simulink model "gmStateSpaceHDL_buck_convert_test1_V2"  (R2025a)
settings: Solver=FixedStepDiscrete  StartTime=0.0  StopTime=0.005  FixedStep=1/40e6  RelTol=1e-3  AbsTol=1e-3
InitFcn:
  | load('C:\Users\bensa\Desktop\PI3_FPGA_BuckConverter\sschdl\buck_convert_test1\stateSpaceParameters.mat');
values from neighbouring files (symbols this model uses):
  stateSpaceParameters_1 =     [stateSpaceParameters.mat]
libraries: hdlsllib x4, hdlssclib x4, simulink x1
CloseFcn:
  | clear stateSpaceParameters_1
settings Model: Creator=bensa  LastModifiedBy=bensa
settings SolverCC: AutoScaleAbsTol=off  AlgebraicLoopSolver=TrustRegion  MaxZcPerStep=1.0
settings OptimizationCC: BlockReduction=off  ConditionallyExecuteInputs=off  DefaultParameterBehavior=Inlined
settings DebuggingCC: AlgebraicLoopMsg=error  SingleTaskRateTransMsg=error  UnconnectedInputMsg=warning  UnconnectedOutputMsg=warning  UnconnectedLineMsg=warning  SymbolicDimsDataTypeCodeGenerationDiagnostic=none
settings HardwareCC: ProdBitPerPointer=32.0  ProdBitPerSizeT=32.0  ProdBitPerPtrDiffT=32.0  ProdLargestAtomicFloat=None  ProdIntDivRoundTo=Undefined  ProdEndianess=Unspecified  ProdWordSize=32.0  ProdHWDeviceType=ASIC/FPGA->ASIC/FPGA  TargetBitPerPointer=64.0  TargetBitPerSizeT=64.0  TargetBitPerPtrDiffT=64.0  TargetLongLongMode=on  TargetIntDivRoundTo=Zero  TargetEndianess=LittleEndian  TargetWordSize=64.0  TargetHWDeviceType=Custom Processor->MATLAB Host Computer  ProdEqTarget=off
settings ModelReferenceCC: EnableRefExpFcnMdlSchedulingChecks=on
settings SFSimCC: CustomCodeUndefinedFunction=UseInterfaceOnly
settings RTWCC: GPUComputeCapability=3.5  DLArmComputeVersion=19.05
settings SimscapeCC: SimscapeLogType=all  SimscapeLogSimulationStatistics=on  SimscapeLogDataHistory=10000.0

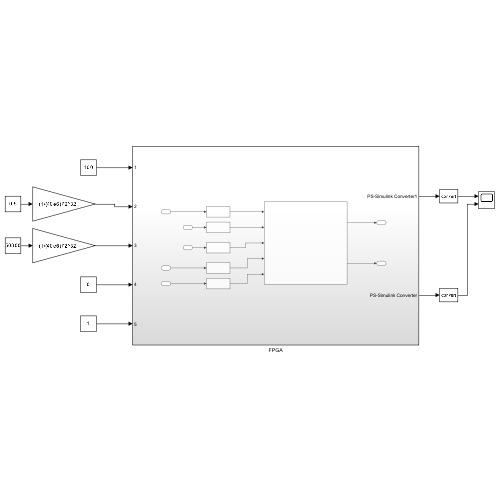
[thumbnail: Simulink's stored preview of the top-level diagram]
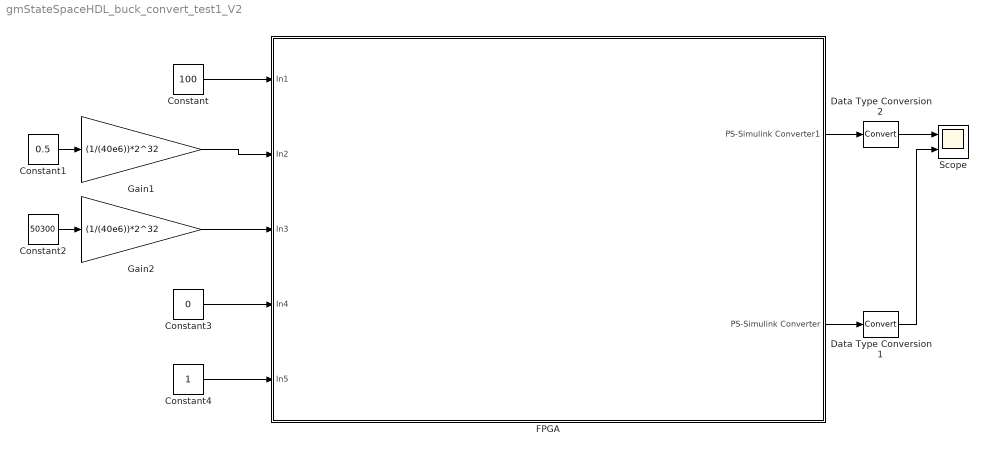
== system gmStateSpaceHDL_buck_convert_test1_V2 ==
  Constant : Constant  Value=100
  Constant1 : Constant  Value=0.5
  Constant2 : Constant  Value=50300
  Constant3 : Constant  Value=0
  Constant4 : Constant
  Data Type Conversion1 : DataTypeConversion  RndMeth=Nearest  SaturateOnIntegerOverflow=off  LockScale=on
  Data Type Conversion2 : DataTypeConversion  RndMeth=Nearest  SaturateOnIntegerOverflow=off  LockScale=on
  FPGA : Subsystem
  Gain1 : Gain  Gain=(1/(40e6))*2^32
  Gain2 : Gain  Gain=(1/(40e6))*2^32
  Scope : Scope  NumInputPorts=2
      settings: ActiveDisplayYMinimum=-1.4999999999999996  ActiveDisplayYMaximum=13.5
  wires:
  Constant3/1 -> FPGA/4(In4)
  Constant/1 -> FPGA/1(In1)
  Constant2/1 -> Gain2/1
  Constant1/1 -> Gain1/1
  Gain1/1 -> FPGA/2(In2)
  Constant4/1 -> FPGA/5(In5)
  Gain2/1 -> FPGA/3(In3)
  FPGA/1(PS-Simulink Converter1) -> Data Type Conversion2/1
  FPGA/2(PS-Simulink Converter) -> Data Type Conversion1/1
  Data Type Conversion2/1 -> Scope/1
  Data Type Conversion1/1 -> Scope/2

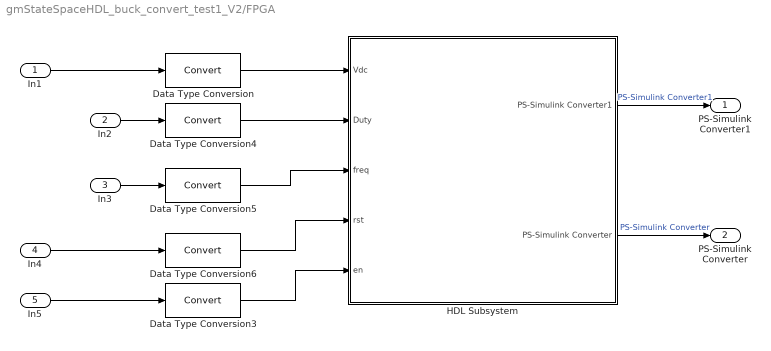
== system gmStateSpaceHDL_buck_convert_test1_V2/FPGA ==
  In1 : Inport
  In2 : Inport  Port=2
  In3 : Inport  Port=3
  In4 : Inport  Port=4
  In5 : Inport  Port=5
  Data Type Conversion{,3..6} (5 alike) : DataTypeConversion  SaturateOnIntegerOverflow=off  RndMeth=Floor
  HDL Subsystem : Subsystem  TreatAsAtomicUnit=on
  PS-Simulink Converter1 : Outport
  PS-Simulink Converter : Outport  Port=2
  wires:
  Data Type Conversion6/1 -> HDL Subsystem/4(rst)
  In2/1 -> Data Type Conversion4/1
  Data Type Conversion4/1 -> HDL Subsystem/2(Duty)
  In5/1 -> Data Type Conversion3/1
  Data Type Conversion/1 -> HDL Subsystem/1(Vdc)
  Data Type Conversion3/1 -> HDL Subsystem/5(en)
  Data Type Conversion5/1 -> HDL Subsystem/3(freq)
  HDL Subsystem/2(PS-Simulink Converter) -> PS-Simulink Converter/1  "PS-Simulink Converter"
  HDL Subsystem/1(PS-Simulink Converter1) -> PS-Simulink Converter1/1  "PS-Simulink Converter1"
  In4/1 -> Data Type Conversion6/1
  In1/1 -> Data Type Conversion/1
  In3/1 -> Data Type Conversion5/1

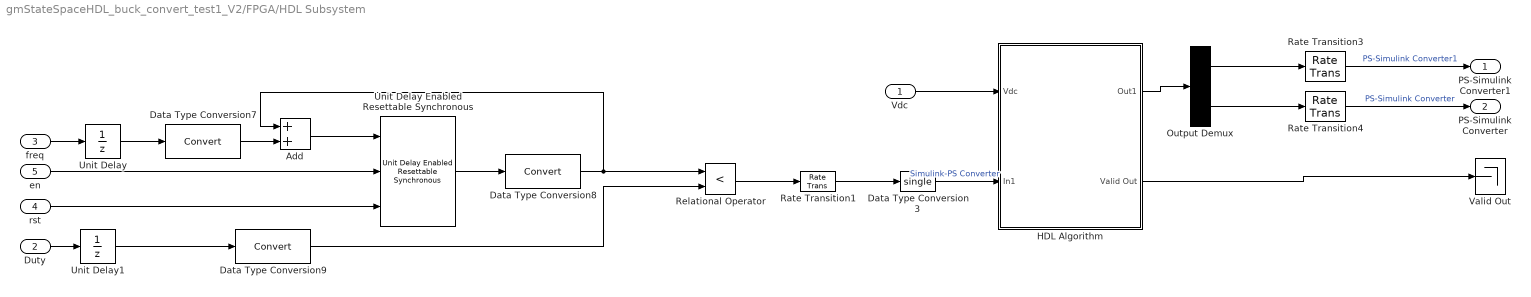
== system gmStateSpaceHDL_buck_convert_test1_V2/FPGA/HDL Subsystem ==
  Vdc : Inport  OutDataTypeStr=uint32
  Duty : Inport  Port=2  OutDataTypeStr=uint32
  freq : Inport  Port=3  OutDataTypeStr=uint32
  rst : Inport  Port=4  OutDataTypeStr=uint32
  en : Inport  Port=5  OutDataTypeStr=uint32
  Add : Sum  OutDataTypeStr=uint32  AccumDataTypeStr=uint32
  Data Type Conversion3 : DataTypeConversion  OutDataTypeStr=single  RndMeth=Nearest  SaturateOnIntegerOverflow=off
  Data Type Conversion7 : DataTypeConversion  SaturateOnIntegerOverflow=off  RndMeth=Floor
  Data Type Conversion8 : DataTypeConversion  SaturateOnIntegerOverflow=off  RndMeth=Floor
  Data Type Conversion9 : DataTypeConversion  SaturateOnIntegerOverflow=off  RndMeth=Floor
  HDL Algorithm : Subsystem
  Output Demux : Demux  Outputs=2
  Rate Transition1 : RateTransition  OutPortSampleTime=1e-06
  Rate Transition3 : RateTransition  OutPortSampleTimeOpt=Multiple of input port sample time  OutPortSampleTimeMultiple=3
  Rate Transition4 : RateTransition  OutPortSampleTimeOpt=Multiple of input port sample time  OutPortSampleTimeMultiple=3
  Relational Operator : RelationalOperator  Operator=<  OutDataTypeStr=boolean  RndMeth=Simplest  InputSameDT=off
  Unit Delay : UnitDelay  SampleTime=-1  HasFrameUpgradeWarning=on
  Unit Delay Enabled Resettable Synchronous : hdlsllib/Discrete/Unit Delay Enabled Resettable Synchronous  InitialCondition=0.0  SampleTime=-1
  Unit Delay1 : UnitDelay  SampleTime=-1  HasFrameUpgradeWarning=on
  Valid Out : Terminator
  PS-Simulink Converter1 : Outport
  PS-Simulink Converter : Outport  Port=2
  wires:
  HDL Algorithm/2(Valid Out) -> Valid Out/1
  Rate Transition4/1 -> PS-Simulink Converter/1  "PS-Simulink Converter"
  Output Demux/1 -> Rate Transition3/1
  Output Demux/2 -> Rate Transition4/1
  Rate Transition3/1 -> PS-Simulink Converter1/1  "PS-Simulink Converter1"
  HDL Algorithm/1(Out1) -> Output Demux/1
  Add/1 -> Unit Delay Enabled Resettable Synchronous/1
  Unit Delay1/1 -> Data Type Conversion9/1
  Unit Delay/1 -> Data Type Conversion7/1
  Data Type Conversion7/1 -> Add/2
  Data Type Conversion8/1 -> Add/1, Relational Operator/1
  Unit Delay Enabled Resettable Synchronous/1 -> Data Type Conversion8/1
  Data Type Conversion9/1 -> Relational Operator/2
  Rate Transition1/1 -> Data Type Conversion3/1
  Data Type Conversion3/1 -> HDL Algorithm/2(In1)  "Simulink-PS Converter"
  freq/1 -> Unit Delay/1
  Duty/1 -> Unit Delay1/1
  en/1 -> Unit Delay Enabled Resettable Synchronous/2
  rst/1 -> Unit Delay Enabled Resettable Synchronous/3
  Vdc/1 -> HDL Algorithm/1(Vdc)
  Relational Operator/1 -> Rate Transition1/1

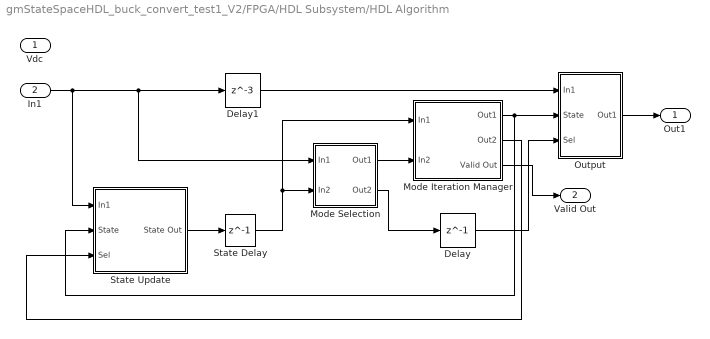
== system gmStateSpaceHDL_buck_convert_test1_V2/FPGA/HDL Subsystem/HDL Algorithm ==
  Vdc : Inport
  In1 : Inport  Port=2
  Delay : Delay  DelayLength=1
  Delay1 : Delay  DelayLength=3
  Mode Iteration Manager : Subsystem
  Mode Selection : Subsystem
  Output : Subsystem
  State Delay : Delay  DelayLength=1  InitialCondition=single(stateSpaceParameters_1.X0)
  State Update : Subsystem
  Out1 : Outport  VectorParamsAs1DForOutWhenUnconnected=off
  Valid Out : Outport  Port=2  VectorParamsAs1DForOutWhenUnconnected=off
  wires:
  In1/1 -> Mode Selection/1(In1), Delay1/1, State Update/1(In1)
  Delay1/1 -> Output/1(In1)
  Mode Iteration Manager/3(Valid Out) -> Valid Out/1
  State Update/1(State Out) -> State Delay/1
  State Delay/1 -> Mode Iteration Manager/1(In1), Mode Selection/2(In2)
  Output/1(Out1) -> Out1/1
  Mode Iteration Manager/1(Out1) -> State Update/2(State), Output/2(State)
  Mode Selection/1(Out1) -> Mode Iteration Manager/2(In2)
  Mode Iteration Manager/2(Out2) -> State Update/3(Sel)
  Mode Selection/2(Out2) -> Delay/1
  Delay/1 -> Output/3(Sel)

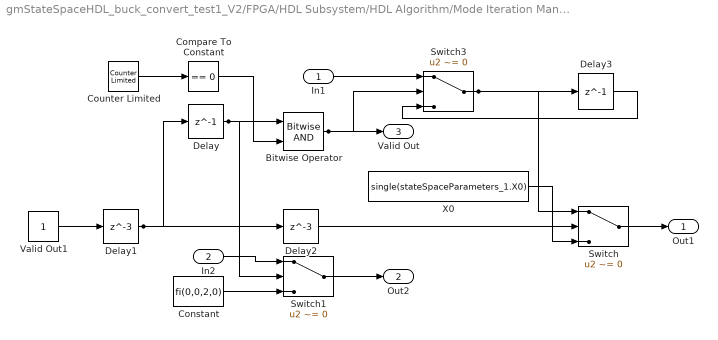
== system gmStateSpaceHDL_buck_convert_test1_V2/FPGA/HDL Subsystem/HDL Algorithm/Mode Iteration Manager ==
  In1 : Inport  LockScale=on
  In2 : Inport  Port=2  OutDataTypeStr=fixdt(0,2,0)  LockScale=on
  Bitwise Operator : simulink/Logic and Bit Operations/Bitwise Operator  logicop=AND  UseBitMask=off  NumInputPorts=2  BitMask=bin2dec('11011001')  BitMaskRealWorld=Stored Integer
      settings: LibrarySourceBlock=|
      | hdlsllib/Logic and Bit
      | Operations/Bitwise
      | Operator
  Compare To Constant : hdlsllib/Logic and Bit Operations/Compare To Constant  relop===  const=0  OutDataTypeStr=boolean
  Constant : Constant  Value=fi(0,0,2,0)  SampleTime=3.333333333333333e-07  LockScale=on
  Counter Limited : hdlsllib/Sources/Counter Limited  uplimit=2  tsamp=-1
  Delay : Delay  DelayLength=1
  Delay1 : Delay  DelayLength=3
  Delay2 : Delay  DelayLength=3
  Delay3 : Delay  DelayLength=1
  Switch : Switch  Criteria=u2 ~= 0  SaturateOnIntegerOverflow=off  InputSameDT=off
  Switch1 : Switch  Criteria=u2 ~= 0  SaturateOnIntegerOverflow=off  InputSameDT=off  OutDataTypeStr=Inherit: Same as first input
      settings: LockScale=on
  Switch3 : Switch  Criteria=u2 ~= 0  SaturateOnIntegerOverflow=off  InputSameDT=off
  Valid Out1 : Constant  OutDataTypeStr=boolean  SampleTime=3.333333333333333e-07
  X0 : Constant  Value=single(stateSpaceParameters_1.X0)  SampleTime=3.333333333333333e-07
  Out1 : Outport  OutDataTypeStr=single  VectorParamsAs1DForOutWhenUnconnected=off
  Out2 : Outport  Port=2  VectorParamsAs1DForOutWhenUnconnected=off
  Valid Out : Outport  Port=3  VectorParamsAs1DForOutWhenUnconnected=off
  wires:
  Valid Out1/1 -> Delay1/1
  Delay1/1 -> Delay2/1, Delay/1
  Counter Limited/1 -> Compare To Constant/1
  Compare To Constant/1 -> Bitwise Operator/2
  In2/1 -> Switch1/1
  In1/1 -> Switch3/1
  Delay/1 -> Switch1/2, Bitwise Operator/1
  Constant/1 -> Switch1/3
  Bitwise Operator/1 -> Valid Out/1, Switch3/2
  Delay2/1 -> Switch/2
  Switch1/1 -> Out2/1
  Switch3/1 -> Delay3/1, Switch/1
  X0/1 -> Switch/3
  Delay3/1 -> Switch3/3
  Switch/1 -> Out1/1

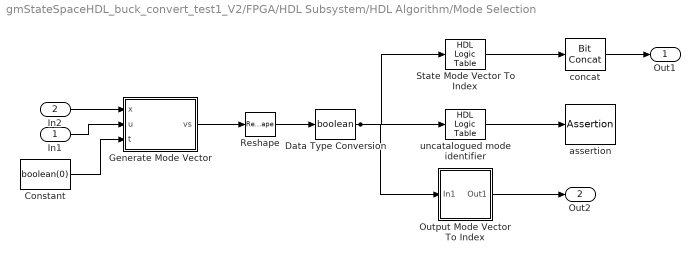
== system gmStateSpaceHDL_buck_convert_test1_V2/FPGA/HDL Subsystem/HDL Algorithm/Mode Selection ==
  In1 : Inport
  In2 : Inport  Port=2  LockScale=on
  Constant : Constant  Value=boolean(0)  SampleTime=3.333333333333333e-07
  Data Type Conversion : DataTypeConversion  OutDataTypeStr=boolean  RndMeth=Nearest  SaturateOnIntegerOverflow=off
  Generate Mode Vector : MATLAB Function  TreatAsAtomicUnit=on
  Output Mode Vector To Index : Subsystem
  Reshape : Reshape
  State Mode Vector To Index : hdlssclib/HDL Logic Table  InputTable=stateSpaceParameters_1.logicTableInput  OutputTable=stateSpaceParameters_1.logicTableOutput
  assertion : Assertion  StopWhenAssertionFail=off
  concat : hdlsllib/Logic and Bit Operations/Bit Concat  numInputs=1
  uncatalogued mode identifier : hdlssclib/HDL Logic Table  InputTable=stateSpaceParameters_1.logicTableInput  OutputTable=ones(size(stateSpaceParameters_1.logicTableOutput,1),1)
  Out1 : Outport  VectorParamsAs1DForOutWhenUnconnected=off  LockScale=on
  Out2 : Outport  Port=2  VectorParamsAs1DForOutWhenUnconnected=off
  wires:
  uncatalogued mode identifier/1 -> assertion/1
  In2/1 -> Generate Mode Vector/1(x)
  In1/1 -> Generate Mode Vector/2(u)
  Reshape/1 -> Data Type Conversion/1
  Output Mode Vector To Index/1(Out1) -> Out2/1
  Data Type Conversion/1 -> State Mode Vector To Index/1, uncatalogued mode identifier/1, Output Mode Vector To Index/1(In1)
  Constant/1 -> Generate Mode Vector/3(t)
  Generate Mode Vector/1(vs) -> Reshape/1
  State Mode Vector To Index/1 -> concat/1
  concat/1 -> Out1/1

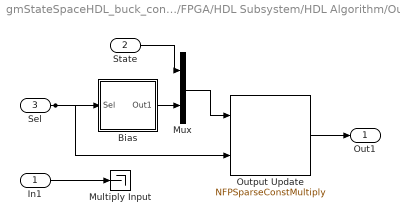
== system gmStateSpaceHDL_buck_convert_test1_V2/FPGA/HDL Subsystem/HDL Algorithm/Output ==
  In1 : Inport
  State : Inport  Port=2
  Sel : Inport  Port=3  LockScale=on
  Bias : Subsystem
  Multiply Input : Terminator
  Mux : Mux  Inputs=2
  Output Update : hdlssclib/NFPSparseConstMultiply  MatrixSource=Dialog  constMatrix=single([stateSpaceParameters_1.Cd repmat(eye(2),[1,1,1])])  MatrixType=single  MatrixSize=[1 1]  ColumnIndices=[1]  RowIndices=[1]  PropDataType=single  defWL=48
  Out1 : Outport  VectorParamsAs1DForOutWhenUnconnected=off
  wires:
  Sel/1 -> Output Update/2, Bias/1(Sel)
  Mux/1 -> Output Update/1
  In1/1 -> Multiply Input/1
  State/1 -> Mux/1
  Bias/1(Out1) -> Mux/2
  Output Update/1 -> Out1/1

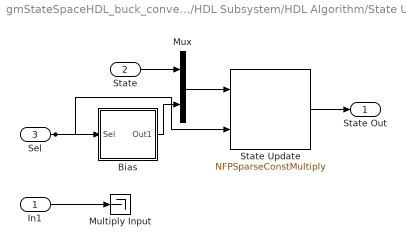
== system gmStateSpaceHDL_buck_convert_test1_V2/FPGA/HDL Subsystem/HDL Algorithm/State Update ==
  In1 : Inport
  State : Inport  Port=2
  Sel : Inport  Port=3  LockScale=on
  Bias : Subsystem
  Multiply Input : Terminator
  Mux : Mux  Inputs=2
  State Update : hdlssclib/NFPSparseConstMultiply  MatrixSource=Dialog  constMatrix=single([stateSpaceParameters_1.Ad repmat(eye(6),[1,1,4])])  MatrixType=single  MatrixSize=[1 1]  ColumnIndices=[1]  RowIndices=[1]  PropDataType=single  defWL=48
  State Out : Outport  OutDataTypeStr=single  VectorParamsAs1DForOutWhenUnconnected=off
  wires:
  Sel/1 -> State Update/2, Bias/1(Sel)
  Bias/1(Out1) -> Mux/2
  In1/1 -> Multiply Input/1
  Mux/1 -> State Update/1
  State/1 -> Mux/1
  State Update/1 -> State Out/1

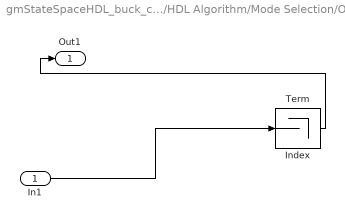
== system gmStateSpaceHDL_buck_convert_test1_V2/FPGA/HDL Subsystem/HDL Algorithm/Mode Selection/Output Mode Vector To Index ==
  In1 : Inport
  Index : Constant  Value=fi(0,0,1,0)  SampleTime=3.333333333333333e-07  LockScale=on
  Term : Terminator
  Out1 : Outport  VectorParamsAs1DForOutWhenUnconnected=off
  wires:
  In1/1 -> Term/1
  Index/1 -> Out1/1

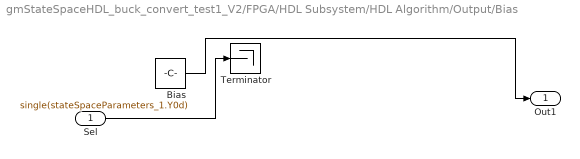
== system gmStateSpaceHDL_buck_convert_test1_V2/FPGA/HDL Subsystem/HDL Algorithm/Output/Bias ==
  Sel : Inport  LockScale=on
  Bias : Constant  Value=single(stateSpaceParameters_1.Y0d)  SampleTime=3.333333333333333e-07
  Terminator : Terminator
  Out1 : Outport  VectorParamsAs1DForOutWhenUnconnected=off
  wires:
  Sel/1 -> Terminator/1
  Bias/1 -> Out1/1

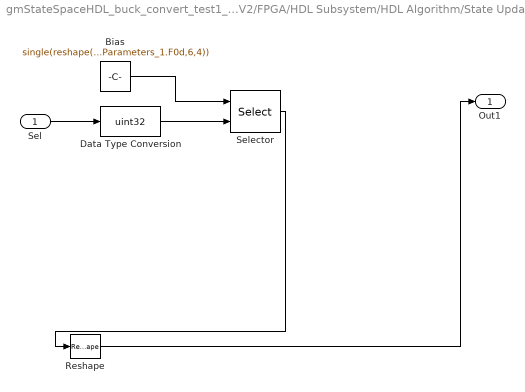
== system gmStateSpaceHDL_buck_convert_test1_V2/FPGA/HDL Subsystem/HDL Algorithm/State Update/Bias ==
  Sel : Inport  LockScale=on
  Bias : Constant  Value=single(reshape(stateSpaceParameters_1.F0d,6,4))  SampleTime=3.333333333333333e-07
  Data Type Conversion : DataTypeConversion  OutDataTypeStr=uint32  RndMeth=Nearest  SaturateOnIntegerOverflow=off
  Reshape : Reshape
  Selector : Selector  NumberOfDimensions=2  IndexMode=Zero-based  InputPortWidth=3  IndexOptions=Select all,Index vector (port)  Indices=[1 3]  OutputSizes=1
  Out1 : Outport  VectorParamsAs1DForOutWhenUnconnected=off
  wires:
  Selector/1 -> Reshape/1
  Bias/1 -> Selector/1
  Sel/1 -> Data Type Conversion/1
  Data Type Conversion/1 -> Selector/2
  Reshape/1 -> Out1/1

== matlab function gmStateSpaceHDL_buck_convert_test1_V2/FPGA/HDL Subsystem/HDL Algorithm/Mode Selection/Generate Mode Vector ==
  data: x input; u input; vs output; t input
function vs = compute_modes(x, u, t)

  tmp1 = (x(6) < (0.0));
  tmp2 = u(1);

  v1 = tmp1;
  v2 = (tmp2 > (2.0));

  vs = [v1 v2];

end
